simulink model "buck_boost"  (R2018a)
settings: Solver=VariableStepAuto  StartTime=0.0  StopTime=0.008  RelTol=1e-3
libraries: powerlib x41
settings Model: Creator=WIN  LastModifiedBy=WIN

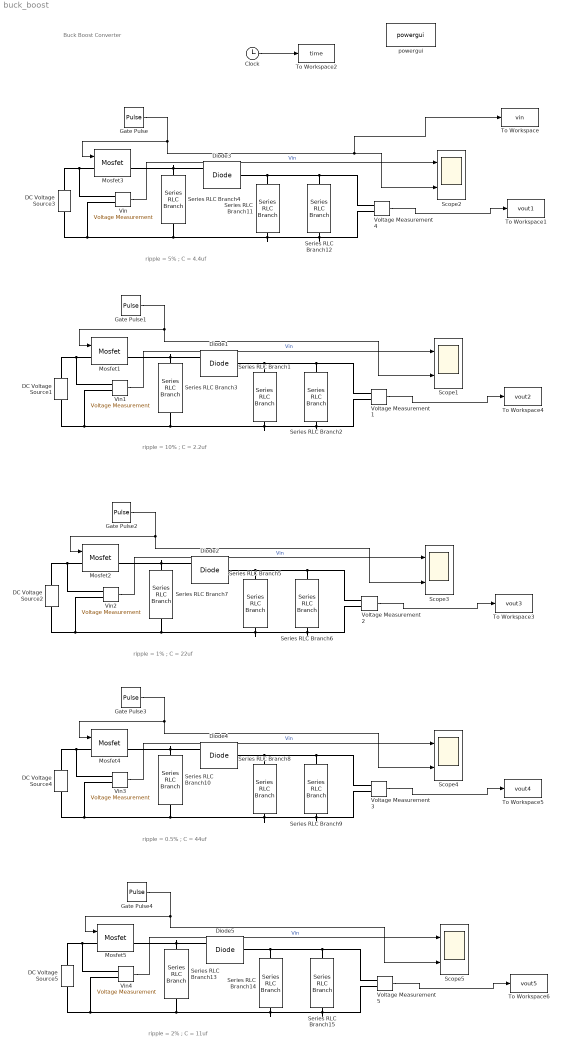
== system buck_boost ==
  note: Buck Boost Converter
  note: ripple = 5% ; C = 4.4uf
  note: ripple = 10% ; C = 2.2uf
  note: ripple = 1% ; C = 22uf
  note: ripple = 0.5% ; C = 44uf
  note: ripple = 2% ; C = 11uf
  Clock : Clock
  DC Voltage Source{1..5} (5 alike) : powerlib/Electrical Sources/DC Voltage Source  Amplitude=20  Measurements=None
  Diode{1..5} (5 alike) : powerlib/Power Electronics/Diode  Ron=0.001  Lon=0  Vf=0.8  IC=0  UseSnubber=0  Rs=500  Cs=250e-9  Measurements=on
  Gate Pulse{,1..4} (5 alike) : DiscretePulseGenerator  PulseType=Time based  Period=1/10000  PulseWidth=33
  Mosfet{1..5} (5 alike) : powerlib/Power Electronics/Mosfet  Ron=0.1  Lon=0  Rd=0.01  Vfd=0  IC=0  Rs=1e5  Cs=inf  Measurements=on
  Scope{1..5} (5 alike) : Scope  NumInputPorts=2
  Series RLC Branch1 : powerlib/Elements/Series RLC Branch  LConnTagsString=__new0  RConnTagsString=__new0  BranchType=C  Resistance=1  Inductance=1e-3  SetiL0=off  InitialCurrent=0  Capacitance=2.2e-6  Setx0=off  InitialVoltage=0  Measurements=None
  Series RLC Branch{3..4,7,10,13} (5 alike) : powerlib/Elements/Series RLC Branch  LConnTagsString=__new0  RConnTagsString=__new0  BranchType=L  Resistance=1  Inductance=4.12e-3  SetiL0=off  InitialCurrent=0  Capacitance=1e-6  Setx0=off  InitialVoltage=0  Measurements=None
  Series RLC Branch11 : powerlib/Elements/Series RLC Branch  LConnTagsString=__new0  RConnTagsString=__new0  BranchType=C  Resistance=1  Inductance=1e-3  SetiL0=off  InitialCurrent=0  Capacitance=4.4e-6  Setx0=off  InitialVoltage=0  Measurements=None
  Series RLC Branch{2,6,9,12,15} (5 alike) : powerlib/Elements/Series RLC Branch  LConnTagsString=__new0  RConnTagsString=__new0  BranchType=R  Resistance=150  Inductance=1e-3  SetiL0=off  InitialCurrent=0  Capacitance=1e-6  Setx0=off  InitialVoltage=0  Measurements=None
  Series RLC Branch14 : powerlib/Elements/Series RLC Branch  LConnTagsString=__new0  RConnTagsString=__new0  BranchType=C  Resistance=1  Inductance=1e-3  SetiL0=off  InitialCurrent=0  Capacitance=11e-6  Setx0=off  InitialVoltage=0  Measurements=None
  Series RLC Branch5 : powerlib/Elements/Series RLC Branch  LConnTagsString=__new0  RConnTagsString=__new0  BranchType=C  Resistance=1  Inductance=1e-3  SetiL0=off  InitialCurrent=0  Capacitance=22e-6  Setx0=off  InitialVoltage=0  Measurements=None
  Series RLC Branch8 : powerlib/Elements/Series RLC Branch  LConnTagsString=__new0  RConnTagsString=__new0  BranchType=C  Resistance=1  Inductance=1e-3  SetiL0=off  InitialCurrent=0  Capacitance=44e-6  Setx0=off  InitialVoltage=0  Measurements=None
  To Workspace : ToWorkspace  VariableName=vin  SampleTime=-1
  To Workspace1 : ToWorkspace  VariableName=vout1  SampleTime=-1
  To Workspace2 : ToWorkspace  VariableName=time  SampleTime=-1
  To Workspace3 : ToWorkspace  VariableName=vout3  SampleTime=-1
  To Workspace4 : ToWorkspace  VariableName=vout2  SampleTime=-1
  To Workspace5 : ToWorkspace  VariableName=vout4  SampleTime=-1
  To Workspace6 : ToWorkspace  VariableName=vout5  SampleTime=-1
  Vin{,1..4} (5 alike) : powerlib/Measurements/Voltage Measurement  PhasorSimulation=off  OutputType=Complex  PSBequivalent=0
  Voltage Measurement{1..5} (5 alike) : powerlib/Measurements/Voltage Measurement  PhasorSimulation=off  OutputType=Complex  PSBequivalent=0
  powergui : powerlib/powergui  Priority=1  SimulationMode=Continuous  SampleTime=50e-6  frequency=60  Iterations=50  frequencyindice=0  Pbase=100e6  ErrMax=1e-4  UnitsV=kV  UnitsW=MW  buscounter=0  FunctionMessages=off  echomessages=off  EnableUseOfTLC=off  CurrentSourceSwitches=off  DisableSnubberDevices=off  DisableRonSwitches=off  DisableVfSwitches=off  DisplayEquations=off  SolverType=Tustin/Backward Euler (TBE)  Interpol=off  ExternalGateDelay=off  methode=off  Ts=100  x0status=blocks  SPID=on  SwTol=0  HookPort=off  RestoreLinks=warning  ResistiveCurrentMeasurement=off  Frange=[0:2:500]  Ylog=off  Xlog=on  ShowGrid=off  save=off  variable=ZData  structure=0  ZoomFFT=off  StartTime=0.0  cycles=1  DisplayStyle=1  fundamental=60  FreqAxis=off  MaxFrequency=1000  frequencyindicesteady=1  RmsSteady=1  display=off
  wires:
  Vin/1 -> Scope2/1  "Vin"
  Gate Pulse/1 -> To Workspace/1, Scope2/2, Mosfet3/1
  Voltage Measurement4/1 -> To Workspace1/1
  Clock/1 -> To Workspace2/1
  Voltage Measurement1/1 -> To Workspace4/1
  Gate Pulse1/1 -> Mosfet1/1, Scope1/2
  Vin1/1 -> Scope1/1  "Vin"
  Vin2/1 -> Scope3/1  "Vin"
  Gate Pulse2/1 -> Scope3/2, Mosfet2/1
  Voltage Measurement2/1 -> To Workspace3/1
  Voltage Measurement3/1 -> To Workspace5/1
  Gate Pulse3/1 -> Mosfet4/1, Scope4/2
  Vin3/1 -> Scope4/1  "Vin"
  Vin4/1 -> Scope5/1  "Vin"
  Gate Pulse4/1 -> Scope5/2, Mosfet5/1
  Voltage Measurement5/1 -> To Workspace6/1
  connections:
  Series RLC Branch11/LConn1 -- Series RLC Branch12/LConn1 -- Voltage Measurement4/LConn1 -- Diode3/LConn1
  Series RLC Branch12/RConn1 -- DC Voltage Source3/LConn1 -- Vin/LConn2 -- Series RLC Branch4/RConn1 -- Series RLC Branch11/RConn1 -- Voltage Measurement4/LConn2
  DC Voltage Source3/RConn1 -- Vin/LConn1 -- Mosfet3/LConn1
  Diode3/RConn1 -- Mosfet3/RConn1 -- Series RLC Branch4/LConn1
  Series RLC Branch2/LConn1 -- Voltage Measurement1/LConn1 -- Series RLC Branch1/LConn1 -- Diode1/LConn1
  Voltage Measurement1/LConn2 -- Series RLC Branch2/RConn1 -- Series RLC Branch1/RConn1 -- Series RLC Branch3/RConn1 -- Vin1/LConn2 -- DC Voltage Source1/LConn1
  Vin1/LConn1 -- DC Voltage Source1/RConn1 -- Mosfet1/LConn1
  Mosfet1/RConn1 -- Diode1/RConn1 -- Series RLC Branch3/LConn1
  Voltage Measurement2/LConn1 -- Diode2/LConn1 -- Series RLC Branch5/LConn1 -- Series RLC Branch6/LConn1
  Series RLC Branch6/RConn1 -- DC Voltage Source2/LConn1 -- Vin2/LConn2 -- Series RLC Branch7/RConn1 -- Series RLC Branch5/RConn1 -- Voltage Measurement2/LConn2
  DC Voltage Source2/RConn1 -- Vin2/LConn1 -- Mosfet2/LConn1
  Diode2/RConn1 -- Mosfet2/RConn1 -- Series RLC Branch7/LConn1
  Diode4/LConn1 -- Voltage Measurement3/LConn1 -- Series RLC Branch9/LConn1 -- Series RLC Branch8/LConn1
  DC Voltage Source4/LConn1 -- Series RLC Branch9/RConn1 -- Voltage Measurement3/LConn2 -- Series RLC Branch8/RConn1 -- Series RLC Branch10/RConn1 -- Vin3/LConn2
  Vin3/LConn1 -- DC Voltage Source4/RConn1 -- Mosfet4/LConn1
  Mosfet4/RConn1 -- Diode4/RConn1 -- Series RLC Branch10/LConn1
  Voltage Measurement5/LConn1 -- Diode5/LConn1 -- Series RLC Branch14/LConn1 -- Series RLC Branch15/LConn1
  Series RLC Branch15/RConn1 -- DC Voltage Source5/LConn1 -- Vin4/LConn2 -- Series RLC Branch13/RConn1 -- Series RLC Branch14/RConn1 -- Voltage Measurement5/LConn2
  DC Voltage Source5/RConn1 -- Vin4/LConn1 -- Mosfet5/LConn1
  Diode5/RConn1 -- Mosfet5/RConn1 -- Series RLC Branch13/LConn1
